simulink model "model_1"  (R2023b)
settings: Solver=VariableStepAuto  StartTime=0.0  StopTime=3.0  RelTol=1e-3
values from neighbouring files (symbols this model uses):
  A = [1,-2,3;2,-3,2;-2,1,-4]    [software_control.m]    (also in task_1.m = [-9,0,-10;-4,-1,-6;6,-2,5]; untitled.m = [-9, 0, -10; -4, -1, -6; 6, -2, 5]; untitled3.m = [-9,0,-10;-4,-1,-6;6,-2,5])
  B = [-3; -1; 3]    [software_control.m]    (also in task_1.m = [0; 0; 0]; untitled.m = [0; 0; 0]; untitled3.m = [0; 0; 0])
settings Model: Creator=dkravchenko  LastModifiedBy=evdokiiagalkina
settings SolverCC: AlgebraicLoopSolver=TrustRegion
settings DebuggingCC: UnconnectedInputMsg=warning  UnconnectedOutputMsg=warning  UnconnectedLineMsg=warning
settings ModelReferenceCC: EnableRefExpFcnMdlSchedulingChecks=on
settings RTWCC: DLArmComputeVersion=19.05

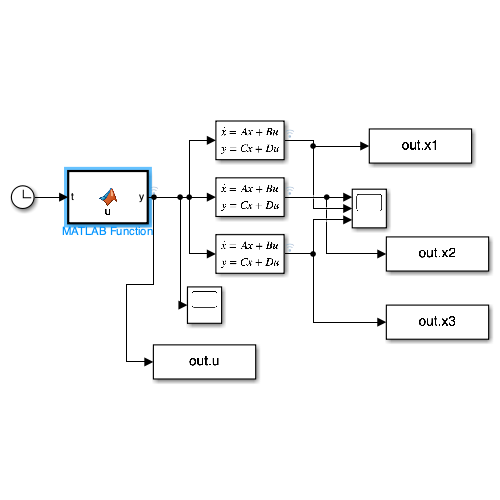
[thumbnail: Simulink's stored preview of the top-level diagram]
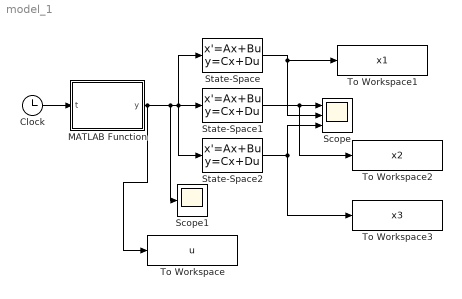
== system model_1 ==
  Clock : Clock
  MATLAB Function : MATLAB Function  TreatAsAtomicUnit=on
  Scope : Scope  NumInputPorts=3
  Scope1 : Scope
  State-Space : StateSpace  A=A  B=B  C=[1, 0, 0]  D=0  InitialCondition=0  ParameterTunability=Optimized  ContinuousStateAttributes='first'
  State-Space1 : StateSpace  A=A  B=B  C=[0, 1, 0]  D=0  InitialCondition=0  ParameterTunability=Unconstrained  ContinuousStateAttributes='second'
  State-Space2 : StateSpace  A=A  B=B  C=[0, 0, 1]  D=0  InitialCondition=0  ContinuousStateAttributes='third'
  To Workspace : ToWorkspace  VariableName=u  SaveFormat=Timeseries  SampleTime=-1
  To Workspace1 : ToWorkspace  VariableName=x1  SaveFormat=Timeseries  SampleTime=-1
  To Workspace2 : ToWorkspace  VariableName=x2  SaveFormat=Timeseries  SampleTime=-1
  To Workspace3 : ToWorkspace  VariableName=x3  SaveFormat=Timeseries  SampleTime=-1
  wires:
  Clock/1 -> MATLAB Function/1(t)
  State-Space/1 -> To Workspace1/1, Scope/2
  State-Space1/1 -> To Workspace2/1, Scope/1
  State-Space2/1 -> To Workspace3/1, Scope/3
  MATLAB Function/1(y) -> To Workspace/1, Scope1/1, State-Space2/1, State-Space/1, State-Space1/1

== matlab function model_1/MATLAB Function ==
  data: t input; y output
function y = u(t)



y = -(140737488355328*exp(2*t - 6)*(20545568074279*cos(t - 3) + 92454691039583*sin(t - 3)))/180718599034703403379736765;
